simulink model "loadcell_model"  (R2024b)
settings: Solver=FixedStepAuto  StartTime=0.0  StopTime=inf  FixedStep=0.01  RelTol=1e-3  EnableMultiTasking=on
libraries: stm32f4xxblockslib x1, simulink x1, dspstat3 x1
settings Model: STM32="{\"AnalogInput\":{\"ID\":\"loadcell_model:23\"}}"  Creator=jirat  LastModifiedBy=jirat
settings OptimizationCC: DefaultParameterBehavior=Inlined  EnhancedBackFolding=on  PassReuseOutputArgsAs=Individual arguments  ZeroExternalMemoryAtStartup=off  ZeroInternalMemoryAtStartup=off  MaxStackSize=512  OptimizeBlockOrder=speed  DifferentSizesBufferReuse=on  OptimizationCustomize=off  EfficientTunableParamExpr=on
settings DebuggingCC: ParameterTunabilityLossMsg=error
settings HardwareCC: ProdBitPerPointer=32  ProdBitPerSizeT=32  ProdBitPerPtrDiffT=32  ProdLargestAtomicInteger=Long  ProdLargestAtomicFloat=Double  ProdWordSize=32  ProdLongLongMode=on  ProdHWDeviceType=ARM Compatible->ARM Cortex-M
settings SFSimCC: MATLABDynamicMemAlloc=off
settings RTWCC: Description=Embedded Coder  SystemTargetFile=ert.tlc  HardwareBoard=STM32G4xx Based  TemplateMakefile=ert_default_tmf  Toolchain=GNU Tools for ARM Embedded Processors
settings CodeAppCC: ForceParamTrailComments=on  IgnoreCustomStorageClasses=off  OperatorAnnotations=on  SimulinkDataObjDesc=on  SFDataObjDesc=on  InsertBlockDesc=on
settings ERTTargetCC: TargetLangStandard=C99 (ISO)  CodeReplacementLibrary=ARM Cortex-M  ExtModeTransport=3  ExtModeStaticAlloc=on  ExtModeStaticAllocSize=2048  ExtModeMexFile=ext_xcp  ExtModeIntrfLevel=Level2 - Open

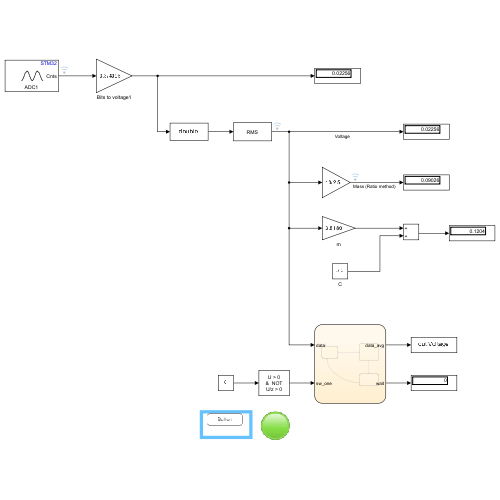
[thumbnail: Simulink's stored preview of the top-level diagram]
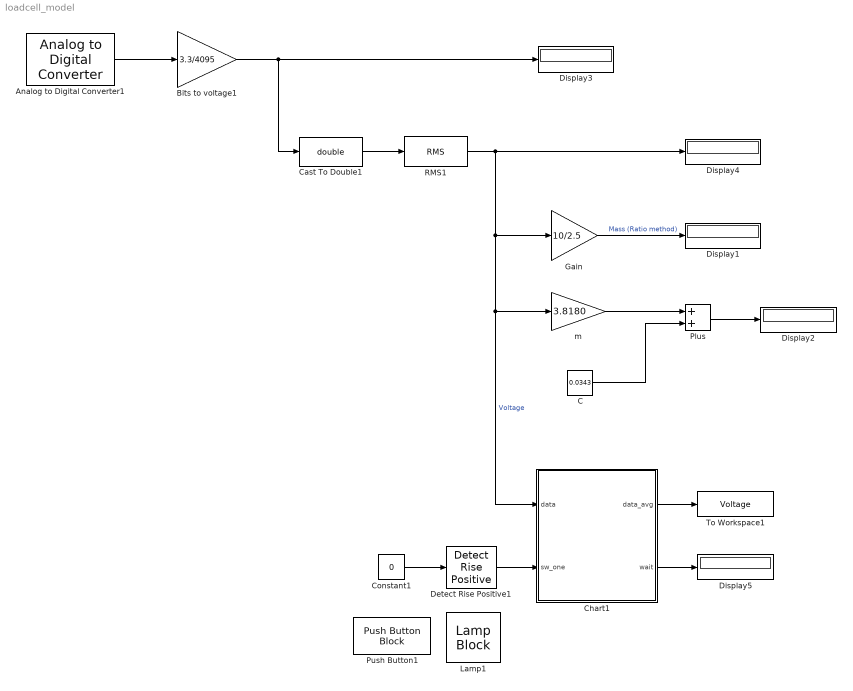
== system loadcell_model ==
  Analog to Digital Converter1 : stm32f4xxblockslib/Analog to Digital Converter  ADCModule=ADC1  ConversionGroup=Regular  TriggerMode=Trigger and read  NumberOfConversions=1  EnableBufferConv=off  BufferLength=1  OutputStatus=off  SampleTime=-1  EnableSimPort=off  hoistedMaskSrc=ECSoC/ECSimCodegen/Analog to Digital Converter
  Bits to voltage1 : Gain  Gain=3.3/4095
  C : Constant  Value=0.0343
  Cast To Double1 : DataTypeConversion  OutDataTypeStr=double  SaturateOnIntegerOverflow=off  RndMeth=Floor
  Chart1 : Stateflow chart  TreatAsAtomicUnit=on
  Constant1 : Constant  Value=0
  Detect Rise Positive1 : simulink/Logic and Bit Operations/Detect Rise Positive  vinit=0  OutDataTypeStr=boolean
  Display{1..5} (5 alike) : Display
  Gain : Gain  Gain=10/2.5
  Lamp1 : LampBlock  LabelPosition=Hide
  Plus : Sum
  Push Button1 : PushButtonBlock  OffValue=0.000000
  RMS1 : dspstat3/RMS  run=off  directionMode=Each column  dimension=1  InputProcessing=Columns as channels (frame based)  reset_popup=None
  To Workspace1 : ToWorkspace  VariableName=Voltage  SampleTime=-1
      settings: Save2DSignal=2-D array (concatenate along first dimension)
  m : Gain  Gain=3.8180
  wires:
  Detect Rise Positive1/1 -> Chart1/2(sw_one)
  RMS1/1 -> m/1, Chart1/1(data), Gain/1, Display4/1  "Voltage"
  Analog to Digital Converter1/1 -> Bits to voltage1/1
  Constant1/1 -> Detect Rise Positive1/1
  Chart1/2(wait) -> Display5/1
  Bits to voltage1/1 -> Cast To Double1/1, Display3/1
  Cast To Double1/1 -> RMS1/1
  Chart1/1(data_avg) -> To Workspace1/1
  Gain/1 -> Display1/1  "Mass (Ratio method)"
  m/1 -> Plus/1
  C/1 -> Plus/2
  Plus/1 -> Display2/1

== stateflow chart loadcell_model/Chart1 ==
  state wait
    entry :
    time = 0
    back = 0
    wait = 1
    during:
    time = time + 0.01
    if time >= 1
    back = 1
    end
  state Init
    sw_one;
    data;
    back = 0
    wait = 0
  state Action
    data_avg = data
  (default) -> Init
  Init -> wait : [sw_one == 1]
  Action -> Init
  wait -> Action : [back == 1]
  data: data input; sw_one input; data_avg output; time local; wait output; back local
